simulink library "downlink_4c2t_lduc_lib"  (Simulink 8.7)
settings: Solver=ode45  StartTime=0.0  StopTime=10.0  RelTol=1e-3
undefined symbols (not defined in the file or in its folder): DUC_LINEUP_param, value
libraries: downlink_4c2t_FoldingCFR_3FIRs_lib x8, DSPBAFilters x4, DSPBAPrim x3, DSPBABase x3, downlink_4c2t_foldingcfr_3firs_lib x1
settings Model: Creator=bigcat  LastModifiedBy=5g

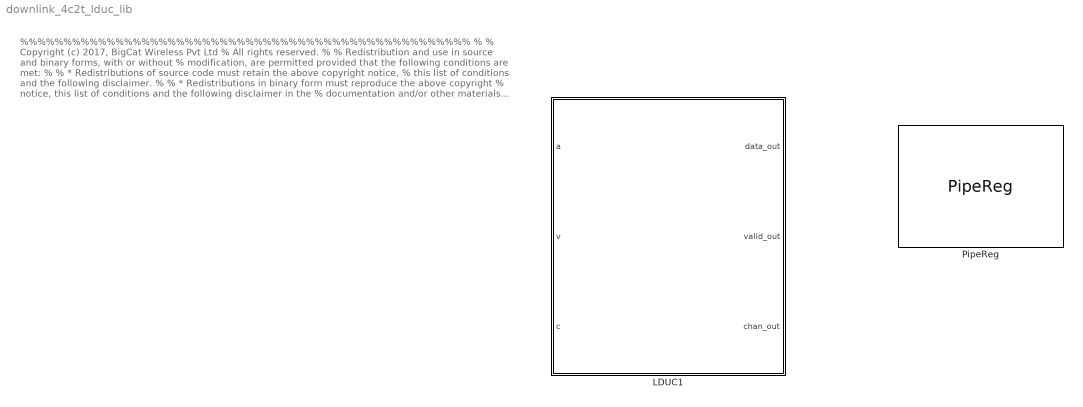
== system downlink_4c2t_lduc_lib ==
  note: %%%%%%%%%%%%%%%%%%%%%%%%%%%%%%%%%%%%%%%%%%%%%%%%%%%%
      |  %
      |  % Copyright (c) 2017, BigCat Wireless Pvt Ltd
      |  % All rights reserved.
      |  %
      |  % Redistribution and use in source and binary forms, with or without
      |  % modification, are permitted provided that the following conditions are met:
      |  %
      |  %     * Redistributions of source code must retain the above copyright notice,
      |  %       this list of conditions and the following disclaimer.
      |  %
      |  %     * Redistributions in binary form must reproduce the above copyright
      |  %       notice, this list of conditions and the following disclaimer in the
      |  %       documentation and/or other materials provided with the distribution.
      |  %
      |  %     * Neither the name of the copyright holder nor the names of its contributors
      |  %       may be used to endorse or promote products derived from this software
      |  %       without specific prior written permission.
      |  %
      |  %
      |  %
      |  % THIS SOFTWARE IS PROVIDED BY THE COPYRIGHT HOLDERS AND CONTRIBUTORS "AS IS"
      |  % AND ANY EXPRESS OR IMPLIED WARRANTIES, INCLUDING, BUT NOT LIMITED TO, THE
      |  % IMPLIED WARRANTIES OF MERCHANTABILITY AND FITNESS FOR A PARTICULAR PURPOSE ARE
      |  % DISCLAIMED. IN NO EVENT SHALL THE COPYRIGHT HOLDER OR CONTRIBUTORS BE LIABLE
      |  % FOR ANY DIRECT, INDIRECT, INCIDENTAL, SPECIAL, EXEMPLARY, OR CONSEQUENTIAL
      |  % DAMAGES (INCLUDING, BUT NOT LIMITED TO, PROCUREMENT OF SUBSTITUTE GOODS OR
      |  % SERVICES; LOSS OF USE, DATA, OR PROFITS; OR BUSINESS INTERRUPTION) HOWEVER
      |  % CAUSED AND ON ANY THEORY OF LIABILITY, WHETHER IN CONTRACT, STRICT LIABILITY,
      |  % OR TORT (INCLUDING NEGLIGENCE OR OTHERWISE) ARISING IN ANY WAY OUT OF THE USE
      |  % OF THIS SOFTWARE, EVEN IF ADVISED OF THE POSSIBILITY OF SUCH DAMAGE.
      |  %
      |   %%%%%%%%%%%%%%%%%%%%%%%%%%%%%%%%%%%%%%%%%%%%%%%%%%%%%
  LDUC1 : Subsystem  mask{clock_margin=0, chan_filter_base_addr=0, hb4_base_addr=0, hb5_base_addr=0, hb5_2_base_addr=0}
      mask prompts: clock_margin "Clock Margin"
      mask Display:
      | disp('LDUC');
      | port_label('input',1,'in_data');
      | port_label('input',2,'in_valid');
      | port_label('input',3,'in_Chan');
      | port_label('output',1,'out_data');
      | port_label('output',2,'out_valid');
      | port_label('output',3,'out_chan');
  PipeReg : downlink_4c2t_foldingcfr_3firs_lib/PipeReg  NPipe=2  Clock_Margin=DUC_LINEUP_param.ClockMargin

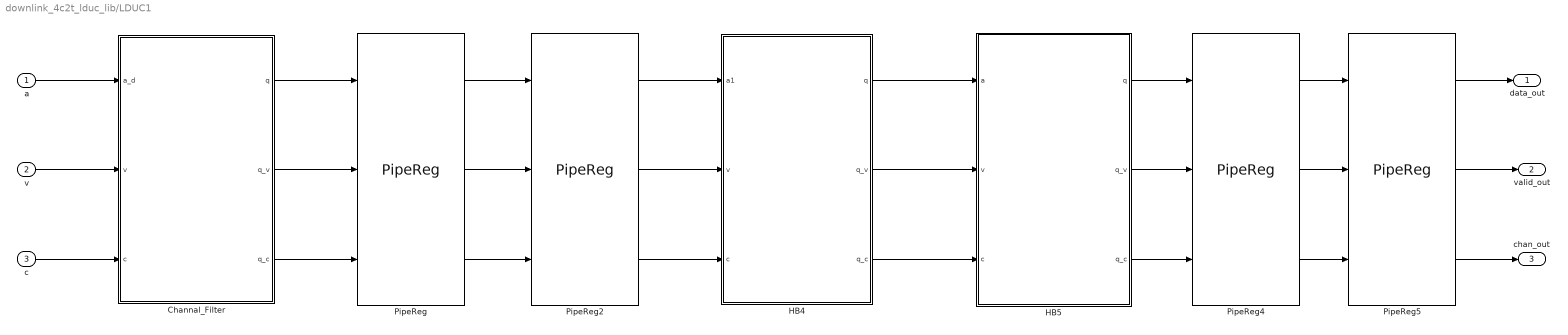
== system downlink_4c2t_lduc_lib/LDUC1 ==
  a : Inport
  v : Inport  Port=2
  c : Inport  Port=3
  Channal_Filter : Subsystem
  HB4 : Subsystem
  HB5 : Subsystem
  PipeReg{,2,4..5} (4 alike) : downlink_4c2t_FoldingCFR_3FIRs_lib/PipeReg  NPipe=2  Clock_Margin=DUC_LINEUP_param.ClockMargin
  data_out : Outport
  valid_out : Outport  Port=2
  chan_out : Outport  Port=3
  wires:
  a/1 -> Channal_Filter/1(a_d)
  v/1 -> Channal_Filter/2(v)
  c/1 -> Channal_Filter/3(c)
  Channal_Filter/3(q_c) -> PipeReg/3
  Channal_Filter/2(q_v) -> PipeReg/2
  Channal_Filter/1(q) -> PipeReg/1
  PipeReg2/1 -> HB4/1(a1)
  PipeReg2/2 -> HB4/2(v)
  PipeReg2/3 -> HB4/3(c)
  PipeReg/3 -> PipeReg2/3
  PipeReg/1 -> PipeReg2/1
  PipeReg/2 -> PipeReg2/2
  HB5/1(q) -> PipeReg4/1
  HB5/2(q_v) -> PipeReg4/2
  HB5/3(q_c) -> PipeReg4/3
  PipeReg4/1 -> PipeReg5/1
  PipeReg4/2 -> PipeReg5/2
  PipeReg4/3 -> PipeReg5/3
  PipeReg5/1 -> data_out/1
  PipeReg5/2 -> valid_out/1
  PipeReg5/3 -> chan_out/1
  HB4/2(q_v) -> HB5/2(v)
  HB4/3(q_c) -> HB5/3(c)
  HB4/1(q) -> HB5/1(a)

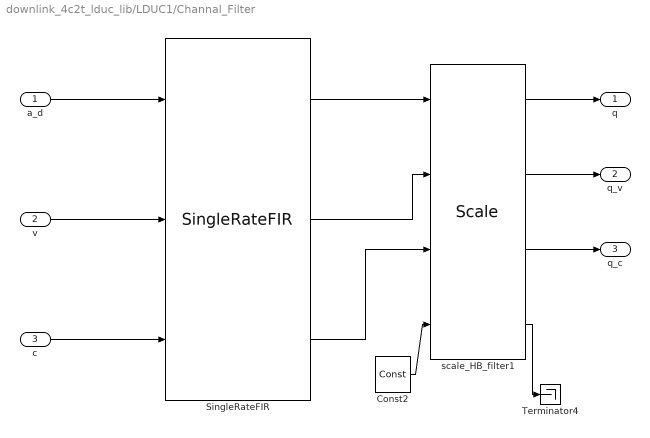
== system downlink_4c2t_lduc_lib/LDUC1/Channal_Filter ==
  a_d : Inport
  v : Inport  Port=2
  c : Inport  Port=3
  Const2 : DSPBAPrim/Const  primtype=const  nInputs=0  nOutputs=1  omode=Inherit via internal rule  otype=sfix(16)  scale=2^-15  rndmethod=Unbiased  factor=1  satmethod=Symmetric  shift_vec=[0 1 2 -1]  value=0  inPortNames=['+'; '+';]  outPortNames=[' ']  dspbaimage=dspba_prim.jpg  text=fprintf('%s', num2str(value));  style=Optimised  visibilities=8 + 1024  floatPrecision=float32_m23  version=20120820
  SingleRateFIR : DSPBAFilters/SingleRateFIR  nInputRate=DUC_LINEUP_param.chan_filter.SampleRate  nchan=DUC_LINEUP_param.chan_filter.ChanCount  symmetry=Symmetrical  coef=DUC_LINEUP_param.chan_filter.coeffs(1,:)  addr=chan_filter_base_addr  rwmode=Read/Write  nband=Use All Taps  latency=4  exposebus=off  version=20090407  recon=off  MM=[0,1,2,3,4,5,6,7,8,9,10,11,12,13,14,15,16,17,18,19]
  Terminator4 : Terminator
  scale_HB_filter1 : DSPBABase/Scale  otype=sfix(DUC_LINEUP_param.output_word_length)  scale=2^-DUC_LINEUP_param.output_fraction_length  rndmethod=Truncate  factor=1  satmethod=Symmetric  shift_vec=0  latency=4  wideSimulation=off  version=20090407
  q : Outport
  q_v : Outport  Port=2
  q_c : Outport  Port=3
  wires:
  scale_HB_filter1/1 -> q/1
  scale_HB_filter1/4 -> Terminator4/1
  a_d/1 -> SingleRateFIR/1
  c/1 -> SingleRateFIR/3
  v/1 -> SingleRateFIR/2
  scale_HB_filter1/3 -> q_c/1
  Const2/1 -> scale_HB_filter1/4
  scale_HB_filter1/2 -> q_v/1
  SingleRateFIR/1 -> scale_HB_filter1/1
  SingleRateFIR/2 -> scale_HB_filter1/2
  SingleRateFIR/3 -> scale_HB_filter1/3

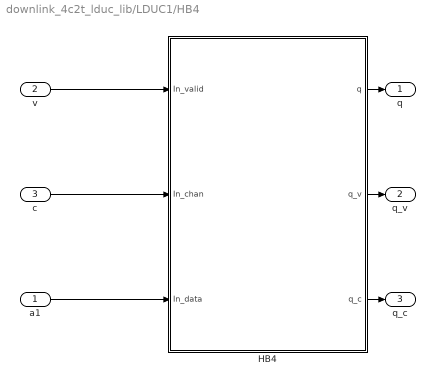
== system downlink_4c2t_lduc_lib/LDUC1/HB4 ==
  a1 : Inport
  v : Inport  Port=2
  c : Inport  Port=3
  HB4 : Subsystem
  q : Outport
  q_v : Outport  Port=2
  q_c : Outport  Port=3
  wires:
  HB4/1(q) -> q/1
  HB4/2(q_v) -> q_v/1
  HB4/3(q_c) -> q_c/1
  a1/1 -> HB4/3(In_data)
  v/1 -> HB4/1(In_valid)
  c/1 -> HB4/2(In_chan)

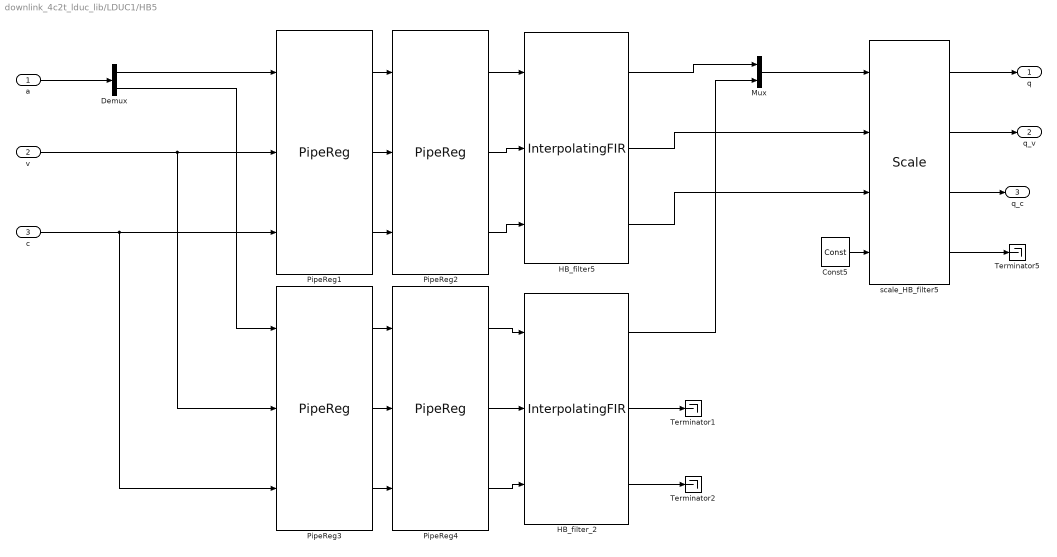
== system downlink_4c2t_lduc_lib/LDUC1/HB5 ==
  a : Inport
  v : Inport  Port=2
  c : Inport  Port=3
  Const5 : DSPBAPrim/Const  primtype=const  nInputs=0  nOutputs=1  omode=Inherit via internal rule  otype=sfix(16)  scale=2^-15  rndmethod=Unbiased  factor=1  satmethod=Symmetric  shift_vec=[0 1 2 -1]  value=0  inPortNames=['+'; '+';]  outPortNames=[' ']  dspbaimage=dspba_prim.jpg  text=fprintf('%s', num2str(value));  style=Optimised  visibilities=8 + 1024  floatPrecision=float32_m23  version=20120820
  Demux : Demux  Outputs=2
  HB_filter5 : DSPBAFilters/InterpolatingFIR  nInputRate=DUC_LINEUP_param.HB_filt5.SampleRate  interp=DUC_LINEUP_param.HB_filt5.Interpolation  nchan=DUC_LINEUP_param.HB_filt5.ChanCount  symmetry=Symmetrical  coef=DUC_LINEUP_param.HB_filt5.coeffs(1,:)  addr=hb5_base_addr  rwmode=Read/Write  nband=Half Band  exposebus=off  latency=10  version=20090407  recon=off  MM=[0,1,2,3,4,5,6,7,8,9,10,11,12,13,14,15]
  HB_filter_2 : DSPBAFilters/InterpolatingFIR  nInputRate=DUC_LINEUP_param.HB_filt5.SampleRate  interp=DUC_LINEUP_param.HB_filt5.Interpolation  nchan=DUC_LINEUP_param.HB_filt5_2.ChanCount  symmetry=Symmetrical  coef=DUC_LINEUP_param.HB_filt5.coeffs(1,:)  addr=hb5_2_base_addr  rwmode=Read/Write  nband=Half Band  exposebus=off  latency=10  version=20090407  recon=off  MM=[0,1,2,3,4,5,6,7,8,9,10,11,12,13,14,15]
  Mux : Mux  Inputs=2
  PipeReg{1..4} (4 alike) : downlink_4c2t_FoldingCFR_3FIRs_lib/PipeReg  NPipe=1  Clock_Margin=DUC_LINEUP_param.ClockMargin
  Terminator1 : Terminator
  Terminator2 : Terminator
  Terminator5 : Terminator
  scale_HB_filter5 : DSPBABase/Scale  otype=sfix(DUC_LINEUP_param.output_word_length)  scale=2^-DUC_LINEUP_param.output_fraction_length  rndmethod=Truncate  factor=1  satmethod=Symmetric  shift_vec=1  latency=4  wideSimulation=off  version=20090407
  q : Outport
  q_v : Outport  Port=2
  q_c : Outport  Port=3
  wires:
  scale_HB_filter5/1 -> q/1
  scale_HB_filter5/3 -> q_c/1
  HB_filter5/3 -> scale_HB_filter5/3
  HB_filter5/2 -> scale_HB_filter5/2
  scale_HB_filter5/2 -> q_v/1
  Const5/1 -> scale_HB_filter5/4
  scale_HB_filter5/4 -> Terminator5/1
  PipeReg1/2 -> PipeReg2/2
  PipeReg1/3 -> PipeReg2/3
  PipeReg1/1 -> PipeReg2/1
  PipeReg2/1 -> HB_filter5/1
  PipeReg2/2 -> HB_filter5/2
  PipeReg2/3 -> HB_filter5/3
  PipeReg4/2 -> HB_filter_2/2
  PipeReg4/3 -> HB_filter_2/3
  PipeReg4/1 -> HB_filter_2/1
  PipeReg3/3 -> PipeReg4/3
  PipeReg3/2 -> PipeReg4/2
  PipeReg3/1 -> PipeReg4/1
  v/1 -> PipeReg3/2, PipeReg1/2
  c/1 -> PipeReg3/3, PipeReg1/3
  HB_filter_2/2 -> Terminator1/1
  HB_filter_2/3 -> Terminator2/1
  a/1 -> Demux/1
  Demux/1 -> PipeReg1/1
  Demux/2 -> PipeReg3/1
  HB_filter5/1 -> Mux/1
  HB_filter_2/1 -> Mux/2
  Mux/1 -> scale_HB_filter5/1

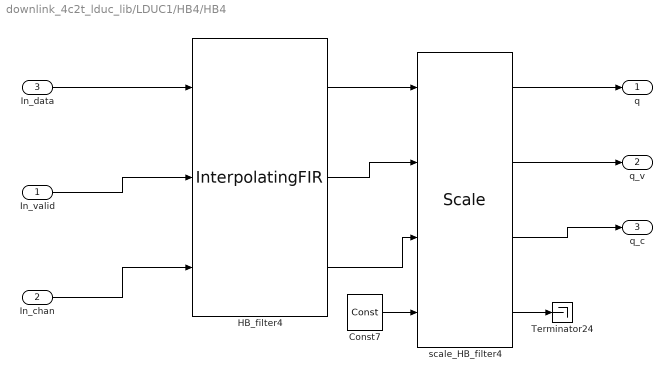
== system downlink_4c2t_lduc_lib/LDUC1/HB4/HB4 ==
  In_valid : Inport
  In_chan : Inport  Port=2
  In_data : Inport  Port=3
  Const7 : DSPBAPrim/Const  primtype=const  nInputs=0  nOutputs=1  omode=Inherit via internal rule  otype=sfix(16)  scale=2^-15  rndmethod=Unbiased  factor=1  satmethod=Symmetric  shift_vec=[0 1 2 -1]  value=0  inPortNames=['+'; '+';]  outPortNames=[' ']  dspbaimage=dspba_prim.jpg  text=fprintf('%s', num2str(value));  style=Optimised  visibilities=8 + 1024  floatPrecision=float32_m23  version=20120820
  HB_filter4 : DSPBAFilters/InterpolatingFIR  nInputRate=DUC_LINEUP_param.HB_filt4.SampleRate  interp=DUC_LINEUP_param.HB_filt4.Interpolation  nchan=DUC_LINEUP_param.HB_filt4.ChanCount  symmetry=Symmetrical  coef=DUC_LINEUP_param.HB_filt4.coeffs(1,:)  addr=hb4_base_addr  rwmode=Read/Write  nband=Half Band  exposebus=off  latency=14  version=20090407  recon=off  MM=[0,1,2,3,4,5,6,7,8,9,10,11,12,13,14,15]
  Terminator24 : Terminator
  scale_HB_filter4 : DSPBABase/Scale  otype=sfix(DUC_LINEUP_param.output_word_length)  scale=2^-DUC_LINEUP_param.output_fraction_length  rndmethod=Truncate  factor=1  satmethod=Symmetric  shift_vec=1  latency=4  wideSimulation=off  version=20090407
  q : Outport
  q_v : Outport  Port=2
  q_c : Outport  Port=3
  wires:
  Const7/1 -> scale_HB_filter4/4
  HB_filter4/3 -> scale_HB_filter4/3
  HB_filter4/2 -> scale_HB_filter4/2
  scale_HB_filter4/1 -> q/1
  HB_filter4/1 -> scale_HB_filter4/1
  scale_HB_filter4/3 -> q_c/1
  In_data/1 -> HB_filter4/1
  scale_HB_filter4/2 -> q_v/1
  scale_HB_filter4/4 -> Terminator24/1
  In_chan/1 -> HB_filter4/3
  In_valid/1 -> HB_filter4/2
